simulink model "BLDC_6step"  (R2020a)
settings: Solver=VariableStepAuto  StartTime=0.0  StopTime=10.0  RelTol=1e-3
InitFcn:
  | BLDC_FOC_Params
values from neighbouring files (symbols this model uses):
  AlignmentDuration = 3 * TimeConstant_s    (= 0.2025)    [BLDC_FOC_Params.m]
  AlignmentDuration_s = 1    [BLDC_FOC_Params.m]
  MotorPolePairs = 4    [BLDC_FOC_Params.m]
  RampupDuration_s = 1    [BLDC_FOC_Params.m]
  RotorInertia_KgM2 = 0.00000011    (= 1.1e-07)    [BLDC_FOC_Params.m]
  Svpwm_freq_hz = 20000    [BLDC_FOC_Params.m]
  Ts = 0.0001    [BLDC_FOC_Params.m]
libraries: ee_lib x21, nesl_utility x12, fl_lib x9, eePwmGenerator x2, simulink x2, eeStairGenerator x1
settings Model: Creator=enzoe  LastModifiedBy=enzoe

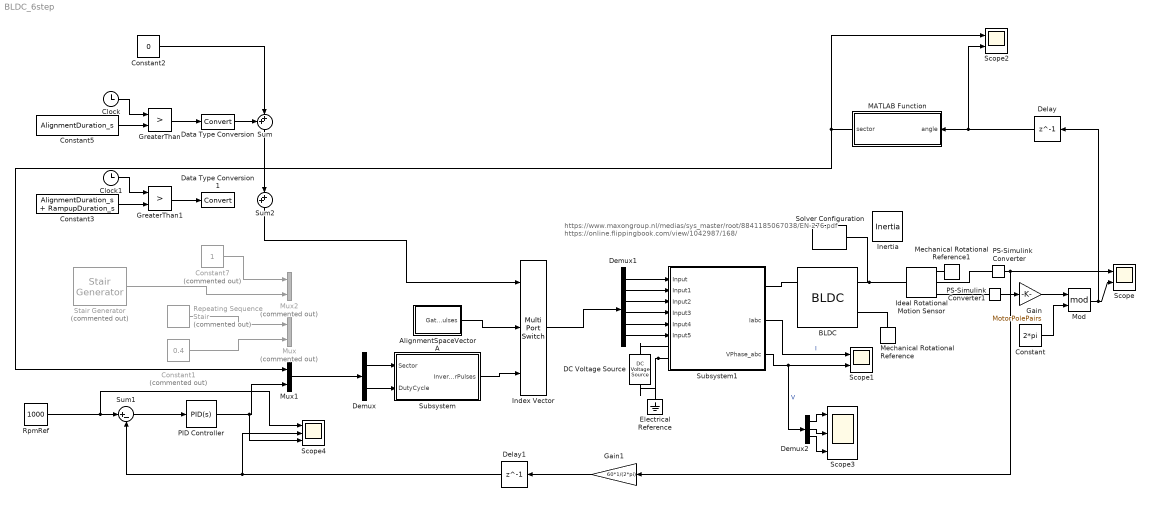
== system BLDC_6step ==
  note: https://www.maxongroup.nl/medias/sys_master/root/8841185067038/EN-276.pdf
      | https://online.flippingbook.com/view/1042987/168/
  AlignmentSpaceVectorA : Subsystem
  BLDC : ee_lib/Electromechanical/Permanent Magnet/BLDC  winding_type=ee.enum.statorconnection.wye  rotor_param=2  pm_flux_linkage=MaximumPermanentMagnetFluxLinkage Wb  theta_constant=pi / (MotorPolePairs*2) rad  emf_max=MaximumRotorInducedBackEmf_V V  DphiDtheta_tab=[0, -.1528, -.1528, .1528, .1528, 0] Wb/rad  back_emf_tab=[0, -9.6, -9.6, 9.6, 9.6, 0] V  rotor_angle_tab=[0, 7.5, 22.5, 37.5, 52.5, 60] deg  w_meas=RotorSpeedUsedForBackEmfMeasurement_RPM rpm  nPolePairs=MotorPolePairs  stator_param=ee.enum.statorparam.LsLmMs  machine_param=ee.enum.dqparameterization.constant  Ld=PhaseInductance H  Lq=PhaseInductance H  idVec=[-200, 0, 200] A  iqVec=[-200, 0, 200] A  LdMatrix=0.00022 * ones(3, 3) H  LqMatrix=0.00022 * ones(3, 3) H  L0=0.00016 H  Ls=PhaseSelfInductance_H H  Lm=StatorInductanceFluctuation_H H  Ms=StatorMutualInductance_H H  Rs=PhaseResistance_Ohm Ohm  zero_sequence=ee.enum.park.zerosequence.include  J=RotorInertia_KgM2 kg*m^2  lam=RotorDamping_NmRads N*m/(rad/s)  axes_param=2  i_d_specify=off  i_d_priority=None  i_d=0 A  i_d_nominal_specify=off  i_d_nominal_unit=A  i_d_nominal_value=1  i_q_specify=off  i_q_priority=None  i_q=0 A  i_q_nominal_specify=off  i_q_nominal_unit=A  i_q_nominal_value=1  torque_specify=off  torque_priority=None  torque=0 N*m  torque_nominal_specify=off  torque_nominal_unit=N*m  torque_nominal_value=1  angular_velocity_specify=off  angular_velocity_priority=High  angular_velocity=0 rpm  angular_velocity_nominal_specify=off  angular_velocity_nominal_unit=rpm  angular_velocity_nominal_value=1  angular_position_specify=off  angular_position_priority=High  angular_position=0 deg  angular_position_nominal_specify=off  angular_position_nominal_unit=deg  angular_position_nominal_value=1  loss_param=ee.enum.ironloss.none  losses_oc=[0, 0, 0] W  losses_sc=[0, 0, 0] W  f_losses=60 Hz  Isc_losses=95 A  Tmeas=298.15 K  alpha=3.93e-3 1/K  alpha_flux=-0.001 1/K  stator_thermal_mass=100 J/K  rotor_thermal_mass=200 J/K  Rm_percent_rotor=90  Rd_percent_rotor=30  temperatureA_specify=off  temperatureA_priority=High  temperatureA=25 degC  temperatureA_nominal_specify=off  temperatureA_nominal_unit=degC  temperatureA_nominal_value=1  temperatureB_specify=off  temperatureB_priority=High  temperatureB=25 degC  temperatureB_nominal_specify=off  temperatureB_nominal_unit=degC  temperatureB_nominal_value=1  temperatureC_specify=off  temperatureC_priority=High  temperatureC=25 degC  temperatureC_nominal_specify=off  temperatureC_nominal_unit=degC  temperatureC_nominal_value=1  temperatureR_specify=off  temperatureR_priority=High  temperatureR=25 degC  temperatureR_nominal_specify=off  temperatureR_nominal_unit=degC  temperatureR_nominal_value=1
      settings: SourceProductBaseCode=PS  InternalSimscapePortConfiguration="{\"Bottom\":[],\"Left\":[{\"id\":\"N\",\"label\":\"~\",\"type\":\"foundation.electrical.three_phase\"},{\"id\":\"n\",\"label\":\"n\",\"type\":\"foundation.electrical.electrical\"}],\"Right\":[{\"id\":\"R\",\"label\":\"R\",\"type\":\"foundation.mechanical.rotational.rotational\"},{\"id\":\"C\",\"label\":\"C\",\"type\":\"foundation.mechanical.rotational.rotational\"}],\"Top\":[]}"
  Clock : Clock
  Clock1 : Clock
  Constant : Constant  Value=2*pi
  Constant1 : Constant  Commented=on  Value=0.4
  Constant2 : Constant  Value=0
  Constant3 : Constant  Value=AlignmentDuration_s + RampupDuration_s
  Constant5 : Constant  Value=AlignmentDuration_s
  Constant7 : Constant  Commented=on
  DC Voltage Source : ee_lib/Additional Components/SPICE Sources/DC Voltage Source  DC=BatteryVoltage V
  Data Type Conversion : DataTypeConversion
  Data Type Conversion1 : DataTypeConversion
  Delay : Delay  DelayLength=1
  Delay1 : Delay  DelayLength=1
  Demux : Demux  Outputs=2
  Demux1 : Demux  Outputs=6
  Demux2 : Demux  Outputs=3
  Electrical Reference : fl_lib/Electrical/Electrical Elements/Electrical Reference
  Gain : Gain  Gain=MotorPolePairs
  Gain1 : Gain  Gain=60*1/(2*pi)
  GreaterThan : RelationalOperator  Operator=>  OutDataTypeStr=boolean  RndMeth=Simplest
  GreaterThan1 : RelationalOperator  Operator=>  OutDataTypeStr=boolean  RndMeth=Simplest
  Ideal Rotational Motion Sensor : fl_lib/Mechanical/Mechanical Sensors/Ideal Rotational Motion Sensor  wrap_angle=simscape.enum.onoff.off  offset=0 rad
  Index Vector : MultiPortSwitch  DataPortOrder=Zero-based contiguous  Inputs=2  zeroidx=on
  Inertia : fl_lib/Mechanical/Rotational Elements/Inertia  inertia=0.0001 kg*m^2  w_specify=off  w_priority=High  w=0 rad/s  w_nominal_specify=off  w_nominal_unit=rad/s  w_nominal_value=1  t_specify=off  t_priority=None  t=0 N*m  t_nominal_specify=off  t_nominal_unit=N*m  t_nominal_value=1
  MATLAB Function : MATLAB Function  TreatAsAtomicUnit=on
  Mechanical Rotational Reference : fl_lib/Mechanical/Rotational Elements/Mechanical Rotational Reference
  Mechanical Rotational Reference1 : fl_lib/Mechanical/Rotational Elements/Mechanical Rotational Reference
  Mod : Math  Operator=mod  SaturateOnIntegerOverflow=on
  Mux : Mux  Commented=on  Inputs=2
  Mux1 : Mux  Inputs=2
  Mux2 : Mux  Commented=on  Inputs=2
  PID Controller : simulink/Continuous/PID Controller  Controller=PID  Form=Parallel  TimeDomain=Continuous-time  UseExternalTs=off  SampleTime=-1  IntegratorMethod=Forward Euler  FilterMethod=Forward Euler  ControllerParametersSource=internal  P=0.01  I=0.01  D=0  UseFilter=on  N=100  TunerSelectOption=Transfer Function Based (PID Tuner App)  InitialConditionSource=internal  InitialConditionForIntegrator=0  InitialConditionForFilter=0  DifferentiatorICPrevScaledInput=0  ExternalReset=none  TrackingMode=off  Kt=1  LimitOutput=off  UpperSaturationLimit=inf  LowerSaturationLimit=-inf  LinearizeAsGain=on  AntiWindupMode=none  Kb=1  POutMin=[]  POutMax=[]  IOutMin=[]  IOutMax=[]  DOutMin=[]  DOutMax=[]  NOutMin=[]  NOutMax=[]  SumOutMin=[]  SumOutMax=[]  SaturationOutMin=[]  SaturationOutMax=[]  PParamMin=[]  PParamMax=[]  IParamMin=[]  IParamMax=[]  DParamMin=[]  DParamMax=[]  NParamMin=[]  NParamMax=[]  KbParamMin=[]  KbParamMax=[]  KtParamMin=[]  KtParamMax=[]  KbOutMin=[]  KbOutMax=[]  KtOutMin=[]  KtOutMax=[]  IntegratorOutMin=[]  IntegratorOutMax=[]  FilterOutMin=[]  FilterOutMax=[]  SumI1OutMin=[]  SumI1OutMax=[]  SumI2OutMin=[]  SumI2OutMax=[]  SumI3OutMin=[]  SumI3OutMax=[]  SumI4OutMin=[]  SumI4OutMax=[]  SumDOutMin=[]  SumDOutMax=[]  DifferentiatorOutMin=[]  DifferentiatorOutMax=[]  FilterDiffOutCoefMin=[]  FilterDiffOutCoefMax=[]  ReciprocalOutMin=[]  ReciprocalOutMax=[]  SumDenOutMin=[]  SumDenOutMax=[]  SumNumOutMin=[]  SumNumOutMax=[]  DivideOutMin=[]  DivideOutMax=[]  UdiffTsProdOutMin=[]  UdiffTsProdOutMax=[]  NTsProdOutMin=[]  NTsProdOutMax=[]  UintegralTsProdOutMin=[]  UintegralTsProdOutMax=[]  UngainTsProdOutMin=[]  UngainTsProdOutMax=[]  IntegratorContinuousStateAttributes=''  IntegratorStateMustResolveToSignalObject=off  IntegratorRTWStateStorageClass=Auto  FilterContinuousStateAttributes=''  FilterStateMustResolveToSignalObject=off  FilterRTWStateStorageClass=Auto  ParallelPVariant=InternalParameters  IdealPVariant=Disabled  IVariant=InternalParameters  DVariant=InternalParameters  IntegratorVariant=Continuous  SatVariant=Disabled  AWVariant=Passthrough  PCopyVariant=Disabled  TRVariant=Disabled  FdbkBlocksVariant=Forward  IdealPFdbkVariant=Disabled  SatFdbkVariant=Disabled  DerivativeFilterVariant=ContFilter  NVariant=InternalParameters  NCopyVariant=Disabled  FilterICVariant=InternalICsFilter  IntegratorICVariant=InternalICs  ExternalResetVariant=Disabled  TRSumVariant=Passthrough  SumFdbkVariant=Disabled  SumVariant=Sum_PID  TsampFilterVariant=InternalTs  TsampNgainVariant=Passthrough  TsampIntegralVariant=Passthrough
  PS-Simulink Converter : nesl_utility/PS-Simulink Converter  PhysicalDomain=network_engine_domain  SubClassName=ps_output  LeftPortType=input  RightPortType=output  PseudoPeriodic=off  Frequencies=[]  Unit=inherit  AffineConversion=off
  PS-Simulink Converter1 : nesl_utility/PS-Simulink Converter  PhysicalDomain=network_engine_domain  SubClassName=ps_output  LeftPortType=input  RightPortType=output  PseudoPeriodic=off  Frequencies=[]  Unit=inherit  AffineConversion=off
  Repeating Sequence Stair : simulink/Sources/Repeating Sequence Stair  Commented=on  OutValues=[1 2 3 4 5 6].'  tsamp=0.01  OutMin=[]  OutMax=[]  OutDataTypeStr=double  OutputDataTypeScalingMode=double  OutDataType=fixdt(0,8)  ConRadixGroup=Best Precision: Vector-wise  OutScaling=2^-12
  RpmRef : Constant  Value=1000
  Scope : Scope  NumInputPorts=2
  Scope1 : Scope  NumInputPorts=2
  Scope2 : Scope  NumInputPorts=2
  Scope3 : Scope  NumInputPorts=3
  Scope4 : Scope  NumInputPorts=3
  Solver Configuration : nesl_utility/Solver Configuration  PhysicalDomain=network_engine_domain  SubClassName=solver  LeftPortType=input  RightPortType=generic  Tones=[]  Harmonics=[]  SimulateNoise=off  Profile=off  UseLocalSampling=off  EnableSwitchedLinearOptims=on  FrequencyDomain=off  UseCCode=off  RelTol=0.001  AbsTol=1e-06  MinStep=1e-09  ToWorkspace=off  RevertToSquareIcSolve=off  NumHomotopyIterations=100  PhasorMode=off  PhasorModeNumHarmonics=1  DoDC=off  ResidualTolerance=1e-09  UseLocalSolver=on  LocalSolverChoice=NE_BACKWARD_EULER_ADVANCER  LocalSolverSampleTime=2e-5  DoFixedCost=on  MaxNonlinIter=4  MaxModeIter=2  LinearAlgebra=auto  EquationFormulation=NE_TIME_EF  DelaysMemoryBudget=1024  AutomaticFiltering=off  FilteringTimeConstant=0.001  PartitionStorageMethod=AS_NEEDED  PartitionMemoryBudget=1024  PartitionMethod=ROBUST
  Stair Generator : eeStairGenerator/Stair Generator  Commented=on  LabelModeActiveChoice=Discrete  TimeInput=[0 AlignmentDuration/3 2*AlignmentDuration/3 AlignmentDuration]  AmplitudeInput=[0 0.2 0.3 0.4]  SampleTime=Ts  RepeatPattern=off  OutDataTypeStr=double
      settings: SourceProductBaseCode=PS
  Subsystem : Subsystem
  Subsystem1 : Subsystem
      settings: PortSchema="{\"entries\":[{\"content\":{\"sides\":[{\"content\":{\"connectorIds\":[\"In1\",\"In2\",\"In3\",\"In4\",\"In5\",\"In6\",\"LConn1\",\"LConn2\"]},\"type\":\"ConnectorPlacement.EquallySpacedRectSide\",\"uuid\":\"4a91dc72-3770-4abf-bed3-c4a9f6b4b65e\"},{\"content\":{\"connectorIds\":[\"RConn1\",\"Out1\",\"Out2\"],\"side\":\"RIGHT\"},\"type\":\"ConnectorPlacement.EquallySpacedRectSide\",\"uuid\":\"c06ed33e-65a1-40a2-85db-2ae3e949e0d2\"},{\"content\":{\"connectorIds\":[],\"side\":\"TOP\"},\"type\":\"ConnectorPlacement.EquallySpacedRectSide\",\"uuid\":\"0b7af1c1-9cb6-4ccc-8dcc-bc330691322d\"}]},\"type\":\"ConnectorPlacement.EquallySpacedConnector\",\"uuid\":\"fc3d9dc5-347b-4e6e-ad3c-0830f77ecff8\"}],\"packageUris\":[\"http://schema.mathworks.com/mf0/Connector/19700101\"],\"version\":\"1.0\"}"
  Sum : Sum  Inputs=++|
  Sum1 : Sum  Inputs=|+-
  Sum2 : Sum  Inputs=++|
  wires:
  Demux1/5 -> Subsystem1/5(Input4)
  Demux1/6 -> Subsystem1/6(Input5)
  Subsystem1/1(Iabc) -> Scope1/1  "I"
  Demux1/4 -> Subsystem1/4(Input3)
  Demux1/1 -> Subsystem1/1(Input)
  Demux1/2 -> Subsystem1/2(Input1)
  Demux1/3 -> Subsystem1/3(Input2)
  Subsystem1/2(VPhase_abc) -> Scope1/2, Demux2/1  "V"
  Mod/1 -> Delay/1, Scope/2
  Constant/1 -> Mod/2
  PS-Simulink Converter1/1 -> Gain/1
  Gain/1 -> Mod/1
  PS-Simulink Converter/1 -> Gain1/1, Scope/1
  MATLAB Function/1(sector) -> Mux1/1, Scope2/1
  Delay/1 -> Scope2/2, MATLAB Function/1(angle)
  Constant1/1 -> Mux/2
  Demux/1 -> Subsystem/1(Sector)
  Demux/2 -> Subsystem/2(DutyCycle)
  Mux1/1 -> Demux/1
  Repeating Sequence Stair/1 -> Mux/1
  Demux2/1 -> Scope3/1
  Demux2/2 -> Scope3/2
  Demux2/3 -> Scope3/3
  Clock/1 -> GreaterThan/1
  Constant5/1 -> GreaterThan/2
  Constant2/1 -> Sum/2
  Data Type Conversion/1 -> Sum/1
  GreaterThan/1 -> Data Type Conversion/1
  Stair Generator/1 -> Mux2/2
  Constant7/1 -> Mux2/1
  RpmRef/1 -> Scope4/1, Sum1/1
  Sum1/1 -> PID Controller/1
  PID Controller/1 -> Scope4/3, Mux1/2
  Gain1/1 -> Delay1/1
  Delay1/1 -> Scope4/2, Sum1/2
  GreaterThan1/1 -> Data Type Conversion1/1
  Clock1/1 -> GreaterThan1/1
  Constant3/1 -> GreaterThan1/2
  Sum/1 -> Sum2/2
  Index Vector/1 -> Demux1/1
  Subsystem/1(InverterPulses) -> Index Vector/3
  Sum2/1 -> Index Vector/1
  AlignmentSpaceVectorA/1(GatePulses) -> Index Vector/2
  connections:
  Subsystem1/LConn2 -- DC Voltage Source/RConn1 -- Electrical Reference/LConn1
  DC Voltage Source/LConn1 -- Subsystem1/LConn1
  BLDC/LConn1 -- Subsystem1/RConn1
  Mechanical Rotational Reference/LConn1 -- BLDC/RConn2
  Ideal Rotational Motion Sensor/RConn2 -- PS-Simulink Converter/LConn1
  PS-Simulink Converter1/LConn1 -- Ideal Rotational Motion Sensor/RConn3
  Ideal Rotational Motion Sensor/RConn1 -- Mechanical Rotational Reference1/LConn1
  Ideal Rotational Motion Sensor/LConn1 -- Solver Configuration/RConn1 -- BLDC/RConn1

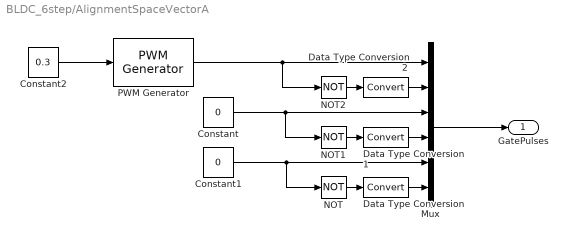
== system BLDC_6step/AlignmentSpaceVectorA ==
  Constant : Constant  Value=0
  Constant1 : Constant  Value=0
  Constant2 : Constant  Value=0.3
  Data Type Conversion : DataTypeConversion
  Data Type Conversion1 : DataTypeConversion
  Data Type Conversion2 : DataTypeConversion
  Mux : Mux  Inputs=6
  NOT : Logic  Operator=NOT  IconShape=distinctive  AllPortsSameDT=off  OutDataTypeStr=boolean
  NOT1 : Logic  Operator=NOT  IconShape=distinctive  AllPortsSameDT=off  OutDataTypeStr=boolean
  NOT2 : Logic  Operator=NOT  IconShape=distinctive  AllPortsSameDT=off  OutDataTypeStr=boolean
  PWM Generator : eePwmGenerator/PWM Generator  CarrCount=Up  Tper=1/Svpwm_freq_hz  Ts=Ts
  GatePulses : Outport
  wires:
  Mux/1 -> GatePulses/1
  NOT1/1 -> Data Type Conversion1/1
  NOT2/1 -> Data Type Conversion2/1
  Constant1/1 -> Mux/5, NOT/1
  Constant/1 -> Mux/3, NOT1/1
  Constant2/1 -> PWM Generator/1
  PWM Generator/1 -> Mux/1, NOT2/1
  NOT/1 -> Data Type Conversion/1
  Data Type Conversion/1 -> Mux/6
  Data Type Conversion1/1 -> Mux/4
  Data Type Conversion2/1 -> Mux/2

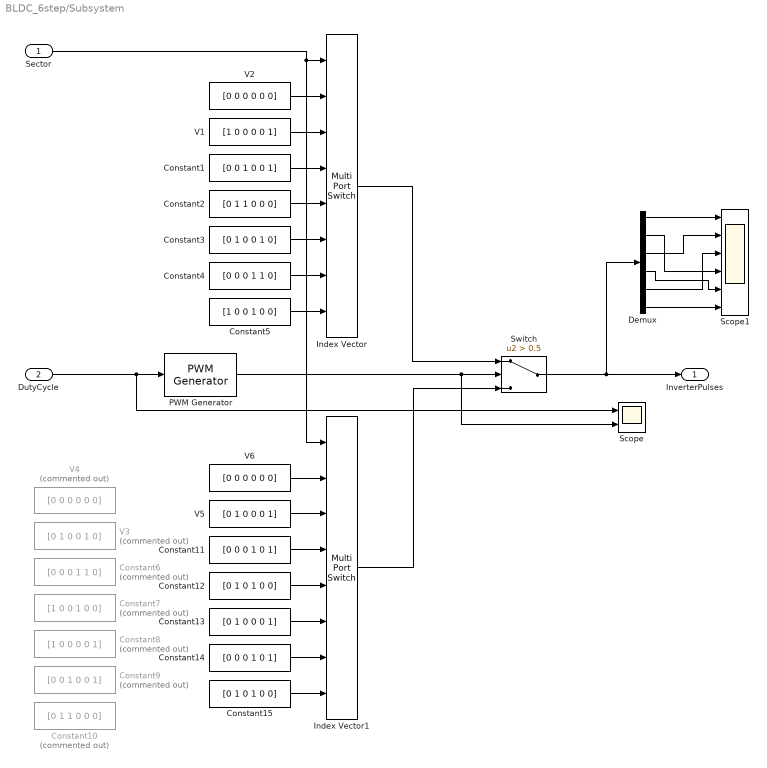
== system BLDC_6step/Subsystem ==
  Sector : Inport
  DutyCycle : Inport  Port=2
  Constant1 : Constant  Value=[0 0 1 0 0 1]
  Constant10 : Constant  Commented=on  Value=[0 1 1 0 0 0]
  Constant11 : Constant  Value=[0 0 0 1 0 1]
  Constant12 : Constant  Value=[0 1 0 1 0 0]
  Constant13 : Constant  Value=[0 1 0 0 0 1]
  Constant14 : Constant  Value=[0 0 0 1 0 1]
  Constant15 : Constant  Value=[0 1 0 1 0 0]
  Constant2 : Constant  Value=[0 1 1 0 0 0]
  Constant3 : Constant  Value=[0 1 0 0 1 0]
  Constant4 : Constant  Value=[0 0 0 1 1 0]
  Constant5 : Constant  Value=[1 0 0 1 0 0]
  Constant6 : Constant  Commented=on  Value=[0 0 0 1 1 0]
  Constant7 : Constant  Commented=on  Value=[1 0 0 1 0 0]
  Constant8 : Constant  Commented=on  Value=[1 0 0 0 0 1]
  Constant9 : Constant  Commented=on  Value=[0 0 1 0 0 1]
  Demux : Demux  Outputs=6
  Index Vector : MultiPortSwitch  DataPortOrder=Zero-based contiguous  Inputs=7  zeroidx=on
  Index Vector1 : MultiPortSwitch  DataPortOrder=Zero-based contiguous  Inputs=7  zeroidx=on
  PWM Generator : eePwmGenerator/PWM Generator  CarrCount=Up  Tper=1/Svpwm_freq_hz  Ts=Ts
  Scope : Scope  NumInputPorts=2
  Scope1 : Scope  NumInputPorts=6
  Switch : Switch  Criteria=u2 > Threshold  Threshold=0.5
  V1 : Constant  Value=[1 0 0 0 0 1]
  V2 : Constant  Value=[0 0 0 0 0 0]
  V3 : Constant  Commented=on  Value=[0 1 0 0 1 0]
  V4 : Constant  Commented=on  Value=[0 0 0 0 0 0]
  V5 : Constant  Value=[0 1 0 0 0 1]
  V6 : Constant  Value=[0 0 0 0 0 0]
  InverterPulses : Outport
  wires:
  V1/1 -> Index Vector/3
  Constant1/1 -> Index Vector/4
  Constant2/1 -> Index Vector/5
  Constant3/1 -> Index Vector/6
  Constant4/1 -> Index Vector/7
  Constant5/1 -> Index Vector/8
  Index Vector/1 -> Switch/1
  Sector/1 -> Index Vector1/1, Index Vector/1
  V2/1 -> Index Vector/2
  DutyCycle/1 -> Scope/1, PWM Generator/1
  PWM Generator/1 -> Scope/2, Switch/2
  Constant12/1 -> Index Vector1/5
  Constant14/1 -> Index Vector1/7
  Constant13/1 -> Index Vector1/6
  Constant11/1 -> Index Vector1/4
  Constant15/1 -> Index Vector1/8
  V6/1 -> Index Vector1/2
  V5/1 -> Index Vector1/3
  Index Vector1/1 -> Switch/3
  Switch/1 -> Demux/1, InverterPulses/1
  Demux/1 -> Scope1/1
  Demux/3 -> Scope1/2
  Demux/5 -> Scope1/3
  Demux/2 -> Scope1/4
  Demux/4 -> Scope1/5
  Demux/6 -> Scope1/6

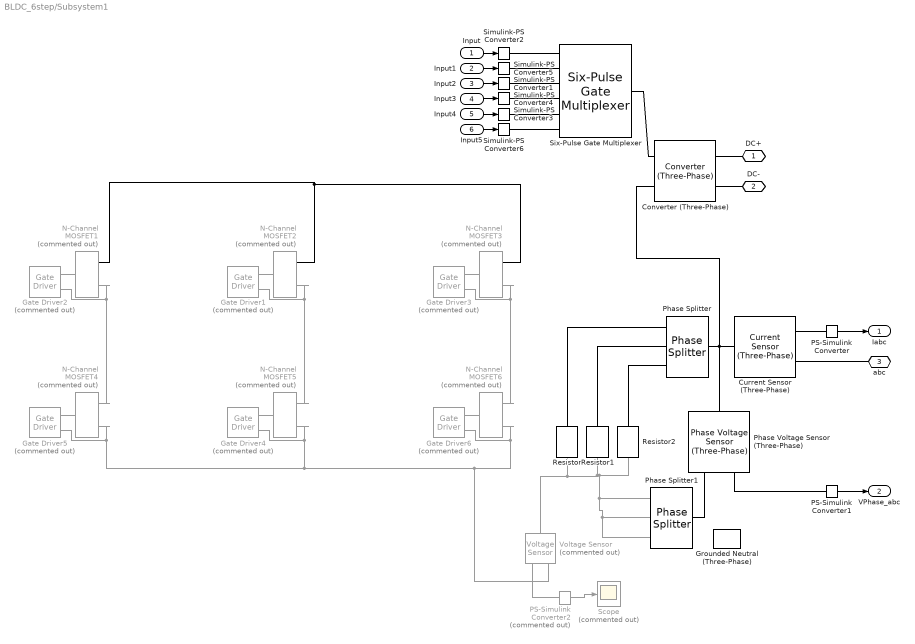
== system BLDC_6step/Subsystem1 ==
  Input : Inport
  Input1 : Inport  Port=2
  Input2 : Inport  Port=3
  Input3 : Inport  Port=4
  Input4 : Inport  Port=5
  Input5 : Inport  Port=6
  Converter (Three-Phase) : ee_lib/Semiconductors & Converters/Converters/Converter (Three-Phase)  device_type=ee.enum.converters.switchingdevice.ideal  Vf=0.8 V  Ron=0.001 Ohm  Rds=0.001 Ohm  Goff=1e-6 1/Ohm  Vth=0.5 V  Vgt=1 V  Vgt_off=-1 V  Ih=1 A  diode_param=ee.enum.converters.protectiondiode.nodynamics  diode_Vf=0.8 V  diode_Ron=0.001 Ohm  diode_Goff=1e-5 1/Ohm  diode_C=50 nF  diode_iRM=-235 A  diode_iF=300 A  diode_idot=-50 A/us  diode_trr_param=ee.enum.converters.diodetrr.trr_factor  diode_trr_factor=3  diode_trr=15 us  diode_Qrr=1500 s*uA  snubber_type=ee.enum.converters.snubber.exclude  Rs=0.1 Ohm  Cs=1e-7 F
      settings: SourceProductBaseCode=PS
  Current Sensor (Three-Phase) : ee_lib/Sensors & Transducers/Current Sensor (Three-Phase)
  Gate Driver{1..6} (6 alike) : ee_lib/Semiconductors & Converters/Gate Driver  Commented=on  vHigh=15 V  vLow=0 V  parameterization=1  rHigh=2 Ohm  rLow=2 Ohm  tRise=20 ns  tFall=20 ns  cLoad=10 nF  enable_faults=0  t_fault=1 s  fault_type=1  uHighValue=0.7  uLowValue=0.3  tHigh=50 ns  tLow=50 ns  ZonTime_specify=off  ZonTime_priority=None  ZonTime=0 s  ZoffTime_specify=off  ZoffTime_priority=None  ZoffTime=0 s  uHigh=2.0 V  uLow=0.8 V
      settings: SourceProductBaseCode=PS  InternalSimscapePortConfiguration="{\"Bottom\":[],\"Left\":[{\"id\":\"u\",\"label\":\"u\",\"type\":\"input\"}],\"Right\":[{\"id\":\"G\",\"label\":\"G\",\"type\":\"foundation.electrical.electrical\"},{\"id\":\"S\",\"label\":\"S\",\"type\":\"foundation.electrical.electrical\"}],\"Top\":[]}"
  Grounded Neutral (Three-Phase) : ee_lib/Connectors & References/Grounded Neutral (Three-Phase)
      settings: SourceProductBaseCode=PS
  N-Channel MOSFET{1..6} (6 alike) : ee_lib/Semiconductors & Converters/N-Channel MOSFET  Commented=on  paramTerminal=ee.enum.mosfet.numberOfTerminals.three  parameterization=ee.enum.parameterization.datasheet  prmDatasheet=ee.enum.temperatureParameterization.none  prmEquCoeff=ee.enum.temperatureParameterization.none  Beta=5.0 A/V^2  Rds=0.025 Ohm  Id=6.0 A  Vgs=10 V  Vth=1.7 V  Vth0=1.7 V  lam=0 1/V  gamma_vth=0.5 V^0.50000  phib=0.5 V  Vth1=1.9071 V  Vbs1=-1 V  Vth2=2.066 V  Vbs2=-2 V  Tmeas=25 degC  RS=0.0001 Ohm  RD=0.01 Ohm  RB=0.001 Ohm  C_param=ee.enum.mosfet.capacitanceParam.fixedciss  C_GS=270 pF  C_GD=80 pF  C_DS=0 pF  C_iss=350 pF  C_rss=80 pF  C_oss=0 pF  charge_linearity_param=ee.enum.mosfet.cgdLinearity.constant  C_OX=200 pF  V_C_OX=-0.5 V  C_iss_vec=[720, 700, 590, 470, 390, 310] pF  C_rss_vec=[450, 400, 300, 190, 95, 55] pF  C_oss_vec=[900, 810, 690, 420, 270, 170] pF  C_GS_vec=[270, 300, 290, 280, 295, 255] pF  C_GD_vec=[450, 400, 300, 190, 95, 55] pF  C_DS_vec=[450, 410, 390, 230, 175, 115] pF  C_Vds_vec=[.1, .3, 1, 3, 10, 30] V  V_GS_for_cap_data=0 V  charge_linearity_param_vgb=ee.enum.mosfet.cgbLinearity.instantly  IsDiode=0 A  Vbi=0.6 V  n=1  Cj0Diode=0 pF  TT=50e-9 s  dVth_dT=-6 mV/K  dVth0_dT=-6 mV/K  Rds_T2=0.037 Ohm  Tmeas2=125 degC  BEXDatasheet=-1.5  BEXEquCoeff=-1.5  etaisDatasheet=3  etaisEquCoeff=3  TdeviceDatasheet=25 degC  TdeviceEquCoeff=25 degC  thermal_network_parameterization=ee.enum.thermalNetworkTopology.cauer  Rth=[0, 10] K/W  Rth_Foster=[4, 6] K/W  thermal_mass_parameterization=ee.enum.thermalNetwork.timeconstant  thermal_mass=[0, 1] J/K  thermal_mass_Foster=[1.5, 3] J/K  thermal_time_constant=[0, 10] s  thermal_time_constant_Foster=[6, 18] s  thermal_mass_initial_temperatures=[25, 25] degC  betaref=18 A/V^2  Vfbref=-1.1 V  gamma=3.5 V^0.50000  phib2ref=1 V  thesatref=0.4 1/V  alpha=0  Vp=5e-2 V  thesrref=0 1/V  m=8  Tref=25 degC  Cox=1500 pF  Cgso=100 pF  Cgdo=14 pF  Rsref=2e-3 Ohm  Rdref=0.17 Ohm  Rgref=8.4 Ohm  Rbref=2e-3 Ohm  Isref=5.2e-13 A  Cj0=480 pF  Tprm=1  etabet=1.3  Stvfb=5e-4 V/K  Stphib=-8.5e-4 V/K  etasat=1.04  etasr=0.65  etar=0.95  etais=3  Tsim=25 degC  T0=[25, 25] degC
  PS-Simulink Converter : nesl_utility/PS-Simulink Converter  PhysicalDomain=network_engine_domain  SubClassName=ps_output  LeftPortType=input  RightPortType=output  PseudoPeriodic=off  Frequencies=[]  Unit=inherit  AffineConversion=off
  PS-Simulink Converter1 : nesl_utility/PS-Simulink Converter  PhysicalDomain=network_engine_domain  SubClassName=ps_output  LeftPortType=input  RightPortType=output  PseudoPeriodic=off  Frequencies=[]  Unit=inherit  AffineConversion=off
  PS-Simulink Converter2 : nesl_utility/PS-Simulink Converter  Commented=on  PhysicalDomain=network_engine_domain  SubClassName=ps_output  LeftPortType=input  RightPortType=output  PseudoPeriodic=off  Frequencies=[]  Unit=inherit  AffineConversion=off
  Phase Splitter : ee_lib/Connectors & References/Phase Splitter
      settings: SourceProductBaseCode=PS
  Phase Splitter1 : ee_lib/Connectors & References/Phase Splitter
      settings: SourceProductBaseCode=PS
  Phase Voltage Sensor (Three-Phase) : ee_lib/Sensors & Transducers/Phase Voltage Sensor (Three-Phase)
      settings: SourceProductBaseCode=PS
  Resistor : fl_lib/Electrical/Electrical Elements/Resistor  R=1000 Ohm  i_specify=off  i_priority=None  i=0 A  i_nominal_specify=off  i_nominal_unit=A  i_nominal_value=1  v_specify=off  v_priority=None  v=0 V  v_nominal_specify=off  v_nominal_unit=V  v_nominal_value=1
  Resistor1 : fl_lib/Electrical/Electrical Elements/Resistor  R=1000 Ohm  i_specify=off  i_priority=None  i=0 A  i_nominal_specify=off  i_nominal_unit=A  i_nominal_value=1  v_specify=off  v_priority=None  v=0 V  v_nominal_specify=off  v_nominal_unit=V  v_nominal_value=1
  Resistor2 : fl_lib/Electrical/Electrical Elements/Resistor  R=1000 Ohm  i_specify=off  i_priority=None  i=0 A  i_nominal_specify=off  i_nominal_unit=A  i_nominal_value=1  v_specify=off  v_priority=None  v=0 V  v_nominal_specify=off  v_nominal_unit=V  v_nominal_value=1
  Scope : Scope  Commented=on
  Simulink-PS Converter{1..6} (6 alike) : nesl_utility/Simulink-PS Converter  PhysicalDomain=network_engine_domain  SubClassName=ps_input  LeftPortType=input  RightPortType=output  PseudoPeriodic=off  Frequencies=[]  NoiseDistribution=none  NoiseParameters=[]  Unit=1  AffineConversion=off  FilteringAndDerivatives=provide  SimscapeFilterOrder=1  InputFilterTimeConstant=0.001  UdotUserProvided=0
  Six-Pulse Gate Multiplexer : ee_lib/Semiconductors & Converters/Converters/Six-Pulse Gate Multiplexer  R=0 Ohm
      settings: SourceProductBaseCode=PS  InternalSimscapePortConfiguration="{\"Bottom\":[],\"Left\":[{\"id\":\"GaH\",\"label\":\"Ga(H)\",\"type\":\"input\"},{\"id\":\"GaL\",\"label\":\"Ga(L)\",\"type\":\"input\"},{\"id\":\"GbH\",\"label\":\"Gb(H)\",\"type\":\"input\"},{\"id\":\"GbL\",\"label\":\"Gb(L)\",\"type\":\"input\"},{\"id\":\"GcH\",\"label\":\"Gc(H)\",\"type\":\"input\"},{\"id\":\"GcL\",\"label\":\"Gc(L)\",\"type\":\"input\"}],\"Right\":[{\"id\":\"p\",\"label\":\"G\",\"type\":\"foundation.electrical.twelve_phase\"}],\"Top\":[]}"
  Voltage Sensor : fl_lib/Electrical/Electrical Sensors/Voltage Sensor  Commented=on
  DC+ : PMIOPort  Side=Left
  DC- : PMIOPort  Port=2  Side=Left
  abc : PMIOPort  Port=3  Side=Right
  Iabc : Outport
  VPhase_abc : Outport  Port=2
  wires:
  Input/1 -> Simulink-PS Converter2/1
  Input1/1 -> Simulink-PS Converter5/1
  Input2/1 -> Simulink-PS Converter1/1
  Input3/1 -> Simulink-PS Converter4/1
  Input4/1 -> Simulink-PS Converter3/1
  Input5/1 -> Simulink-PS Converter6/1
  PS-Simulink Converter/1 -> Iabc/1
  PS-Simulink Converter1/1 -> VPhase_abc/1
  PS-Simulink Converter2/1 -> Scope/1
  connections:
  N-Channel MOSFET1/LConn1 -- Gate Driver2/RConn1
  N-Channel MOSFET4/RConn1 -- N-Channel MOSFET1/RConn2 -- Gate Driver2/RConn2
  Phase Splitter/RConn2 -- Resistor1/LConn1
  N-Channel MOSFET2/LConn1 -- Gate Driver1/RConn1
  N-Channel MOSFET3/LConn1 -- Gate Driver3/RConn1
  N-Channel MOSFET6/RConn1 -- N-Channel MOSFET3/RConn2 -- Gate Driver3/RConn2
  N-Channel MOSFET6/LConn1 -- Gate Driver6/RConn1
  N-Channel MOSFET4/RConn2 -- Voltage Sensor/RConn2 -- N-Channel MOSFET6/RConn2 -- Gate Driver6/RConn2 -- N-Channel MOSFET5/RConn2 -- Gate Driver4/RConn2 -- Gate Driver5/RConn2
  N-Channel MOSFET5/LConn1 -- Gate Driver4/RConn1
  N-Channel MOSFET4/LConn1 -- Gate Driver5/RConn1
  N-Channel MOSFET1/RConn1 -- N-Channel MOSFET3/RConn1 -- N-Channel MOSFET2/RConn1
  Current Sensor (Three-Phase)/RConn2 -- abc/RConn1
  Phase Voltage Sensor (Three-Phase)/LConn1 -- Converter (Three-Phase)/LConn2 -- Phase Splitter/LConn1 -- Current Sensor (Three-Phase)/LConn1
  PS-Simulink Converter/LConn1 -- Current Sensor (Three-Phase)/RConn1
  PS-Simulink Converter1/LConn1 -- Phase Voltage Sensor (Three-Phase)/RConn1
  Voltage Sensor/LConn1 -- Resistor/RConn1 -- Phase Splitter1/RConn3 -- Phase Splitter1/RConn2 -- Phase Splitter1/RConn1 -- Resistor2/RConn1 -- Resistor1/RConn1
  PS-Simulink Converter2/LConn1 -- Voltage Sensor/RConn1
  DC+/RConn1 -- Converter (Three-Phase)/RConn1
  DC-/RConn1 -- Converter (Three-Phase)/RConn2
  Simulink-PS Converter2/RConn1 -- Six-Pulse Gate Multiplexer/LConn1
  Simulink-PS Converter5/RConn1 -- Six-Pulse Gate Multiplexer/LConn2
  Simulink-PS Converter1/RConn1 -- Six-Pulse Gate Multiplexer/LConn3
  Simulink-PS Converter4/RConn1 -- Six-Pulse Gate Multiplexer/LConn4
  Simulink-PS Converter3/RConn1 -- Six-Pulse Gate Multiplexer/LConn5
  Simulink-PS Converter6/RConn1 -- Six-Pulse Gate Multiplexer/LConn6
  Six-Pulse Gate Multiplexer/RConn1 -- Converter (Three-Phase)/LConn1
  Resistor/LConn1 -- Phase Splitter/RConn1
  N-Channel MOSFET2/RConn2 -- N-Channel MOSFET5/RConn1 -- Gate Driver1/RConn2
  Phase Splitter/RConn3 -- Resistor2/LConn1
  Phase Splitter1/LConn1 -- Phase Voltage Sensor (Three-Phase)/RConn2

== matlab function BLDC_6step/MATLAB Function ==
  data: angle input; sector output
function sector = angleToSector(angle)

if(11*pi/6 < angle || angle <= pi/6)
    sector = 1;
elseif(pi/6 < angle && angle <= 3*pi/6)
    sector = 2;
elseif(3*pi/6 < angle && angle <= 5*pi/6)
    sector = 3;
elseif(5*pi/6 < angle && angle <= 7*pi/6)
    sector = 4;
elseif(7*pi/6 < angle && angle <= 9*pi/6)
    sector = 5;
elseif(9*pi/6 < angle && angle <= 11*pi/6)
    sector = 6;
else
    sector = 0;
    
end
